simulink model "1_spwm"  (R2024b)
settings: Solver=VariableStepDiscrete  StartTime=0.0  StopTime=0.04  RelTol=1e-3
libraries: simulink x1, spsTriangleGeneratorLib x1
settings Model: Creator=vasudha  LastModifiedBy=vasudha

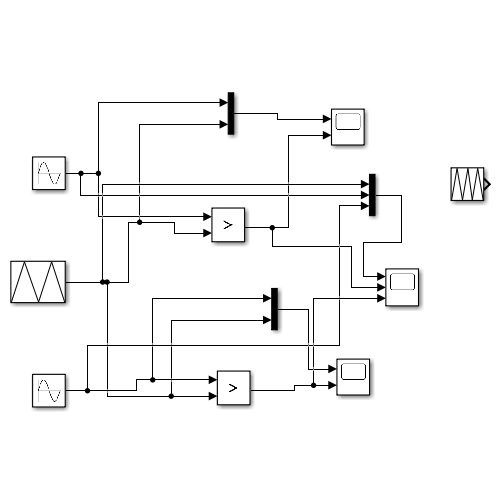
[thumbnail: Simulink's stored preview of the top-level diagram]
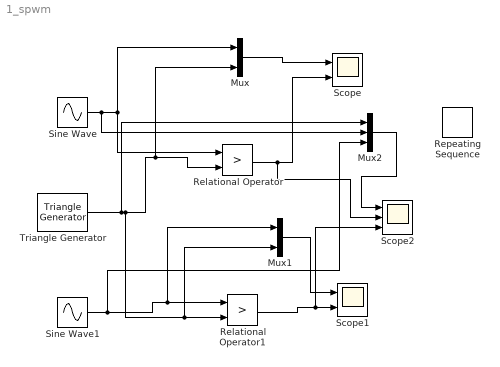
== system 1_spwm ==
  Mux : Mux  Inputs=2
  Mux1 : Mux  Inputs=2
  Mux2 : Mux  Inputs=3
  Relational Operator : RelationalOperator  Operator=>  OutDataTypeStr=boolean  RndMeth=Simplest  InputSameDT=off
  Relational Operator1 : RelationalOperator  Operator=>  OutDataTypeStr=boolean  RndMeth=Simplest  InputSameDT=off
  Repeating Sequence : simulink/Sources/Repeating Sequence  rep_seq_t=[0 0.5e-3 1e-3]  rep_seq_y=[-1 1 -1]
  Scope : Scope  NumInputPorts=2
  Scope1 : Scope  NumInputPorts=2
  Scope2 : Scope  NumInputPorts=3
  Sine Wave : Sin  Frequency=314  SampleTime=0
  Sine Wave1 : Sin  Frequency=314  Phase=3.14  SampleTime=0
  Triangle Generator : spsTriangleGeneratorLib/Triangle Generator  Freq=0.25e3  Phase=0  Ts=0
  wires:
  Sine Wave/1 -> Mux2/2, Mux/1, Relational Operator/1
  Triangle Generator/1 -> Mux2/1, Mux/2, Relational Operator/2, Mux1/2, Relational Operator1/2
  Mux/1 -> Scope/1
  Relational Operator/1 -> Scope2/2, Scope/2
  Sine Wave1/1 -> Mux2/3, Mux1/1, Relational Operator1/1
  Mux1/1 -> Scope1/1
  Relational Operator1/1 -> Scope2/3, Scope1/2
  Mux2/1 -> Scope2/1
